simulink model "CruiseCtrl_StateFeedback_v2"  (R2020a)
settings: Solver=VariableStepAuto  StartTime=0.0  StopTime=40.0  MaxStep=0.001  RelTol=1e-3
values from neighbouring files (symbols this model uses):
  B1 = [B H]    [Driveline_ctrl_design.m]
undefined symbols (not defined in the file or in its folder): A, C1, D1, g, K, kr, teta, ue, x1e, x2e
settings Model: Creator=juan  LastModifiedBy=juan

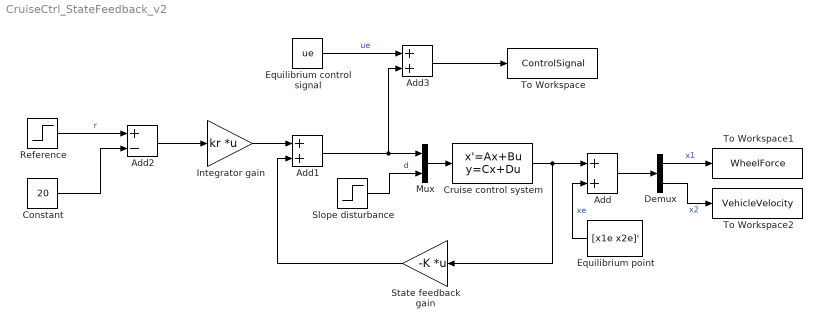
== system CruiseCtrl_StateFeedback_v2 ==
  Add : Sum
  Add1 : Sum
  Add2 : Sum  Inputs=+-
  Add3 : Sum
  Constant : Constant  Value=20
  Cruise control system : StateSpace  A=A  B=B1  C=C1  D=D1
  Demux : Demux  Outputs=2
  Equilibrium control signal : Constant  Value=ue
  "Equilibrium point " : Constant  Value=[x1e x2e]'
  Integrator gain : Gain  Gain=kr  Multiplication=Matrix(K*u)
  Mux : Mux  Inputs=2
  Reference : Step  Before=20  After=25  SampleTime=0
  Slope disturbance : Step  Time=20  After=g*sin(teta)  SampleTime=0
  State feedback gain : Gain  Gain=-K  Multiplication=Matrix(K*u)
  To Workspace : ToWorkspace  VariableName=ControlSignal  SaveFormat=Structure With Time  SampleTime=-1
  To Workspace1 : ToWorkspace  VariableName=WheelForce  SaveFormat=Structure With Time  SampleTime=-1
  To Workspace2 : ToWorkspace  VariableName=VehicleVelocity  SaveFormat=Structure With Time  SampleTime=-1
  wires:
  Demux/1 -> To Workspace1/1  "x1"
  Mux/1 -> Cruise control system/1
  Slope disturbance/1 -> Mux/2  "d"
  Demux/2 -> To Workspace2/1  "x2"
  Cruise control system/1 -> State feedback gain/1, Add/1
  "Equilibrium point "/1 -> Add/2  "xe"
  Add/1 -> Demux/1
  Integrator gain/1 -> Add1/1
  State feedback gain/1 -> Add1/2
  Add1/1 -> Add3/2, Mux/1
  Reference/1 -> Add2/1  "r"
  Add2/1 -> Integrator gain/1
  Constant/1 -> Add2/2
  Equilibrium control signal/1 -> Add3/1  "ue"
  Add3/1 -> To Workspace/1
